simulink model "case8"  (R2024b)
settings: Solver=FixedStepAuto  StartTime=0  StopTime=1  FixedStep=1e-7  RelTol=1e-3
values from neighbouring files (symbols this model uses):
  SG_D_1_D = 0.01056    [IEEE9_case_parameters.m]    (also in case1_parameters.m; case2_parameters.m; case3_parameters.m; case4_parameters.m)
  SG_D_1_EnableSaturation = 0    [IEEE9_case_parameters.m]    (also in case1_parameters.m; case2_parameters.m; case3_parameters.m; case4_parameters.m)
  SG_D_1_f0 = 60    [IEEE9_case_parameters.m]    (also in case1_parameters.m; case2_parameters.m; case3_parameters.m; case4_parameters.m)
  SG_D_1_H = 7.5    [IEEE9_case_parameters.m]    (also in case1_parameters.m; case2_parameters.m; case3_parameters.m; case4_parameters.m)
  SG_D_1_K_A = 20    [IEEE9_case_parameters.m]    (also in case1_parameters.m; case2_parameters.m; case3_parameters.m; case4_parameters.m)
  SG_D_1_K_E = 1.000000e+1    (= 10)    [IEEE9_case_parameters.m]    (also in case1_parameters.m; case2_parameters.m; case3_parameters.m; case4_parameters.m)
  SG_D_1_K_F = 2.363    [IEEE9_case_parameters.m]    (also in case1_parameters.m; case2_parameters.m; case3_parameters.m; case4_parameters.m)
  SG_D_1_K_s = 0.5    [IEEE9_case_parameters.m]    (also in case1_parameters.m = 5; case2_parameters.m = 5; case3_parameters.m = 5; case4_parameters.m = 5)
  SG_D_1_R_a = 0.001088    [IEEE9_case_parameters.m]    (also in case1_parameters.m; case2_parameters.m; case3_parameters.m; case4_parameters.m)
  SG_D_1_S_A = 1    [IEEE9_case_parameters.m]    (also in case1_parameters.m; case2_parameters.m; case3_parameters.m; case4_parameters.m)
  SG_D_1_S_B = 0.103    [IEEE9_case_parameters.m]    (also in case1_parameters.m; case2_parameters.m; case3_parameters.m; case4_parameters.m)
  SG_D_1_S_N = 10.659857    [IEEE9_case_parameters.m]    (also in case1_parameters.m; case2_parameters.m; case3_parameters.m; case4_parameters.m)
  SG_D_1_SpeedPara = 200    [IEEE9_case_parameters.m]    (also in case1_parameters.m; case2_parameters.m; case3_parameters.m; case4_parameters.m)
  SG_D_1_T_0 = 0.720173    [IEEE9_case_parameters.m]    (also in case1_parameters.m = 0.755522; case2_parameters.m = 0.808931; case3_parameters.m = 0.869402; case4_parameters.m = 0.729316)
  SG_D_1_T_1 = 0.3    [IEEE9_case_parameters.m]    (also in case1_parameters.m; case2_parameters.m; case3_parameters.m; case4_parameters.m)
  SG_D_1_T_2 = 0.05    [IEEE9_case_parameters.m]    (also in case1_parameters.m; case2_parameters.m; case3_parameters.m; case4_parameters.m)
  SG_D_1_T_3 = 0.02    [IEEE9_case_parameters.m]    (also in case1_parameters.m; case2_parameters.m; case3_parameters.m; case4_parameters.m)
  SG_D_1_T_4 = 0.005    [IEEE9_case_parameters.m]    (also in case1_parameters.m; case2_parameters.m; case3_parameters.m; case4_parameters.m)
  SG_D_1_T_A = 0.02    [IEEE9_case_parameters.m]    (also in case1_parameters.m; case2_parameters.m; case3_parameters.m; case4_parameters.m)
  SG_D_1_T_dd = 8.000000e+0    (= 8)    [IEEE9_case_parameters.m]    (also in case1_parameters.m; case2_parameters.m; case3_parameters.m; case4_parameters.m)
  SG_D_1_T_ddd = 0.04    [IEEE9_case_parameters.m]    (also in case1_parameters.m; case2_parameters.m; case3_parameters.m; case4_parameters.m)
  SG_D_1_T_E = 0.314    [IEEE9_case_parameters.m]    (also in case1_parameters.m; case2_parameters.m; case3_parameters.m; case4_parameters.m)
  SG_D_1_T_F = 0.35    [IEEE9_case_parameters.m]    (also in case1_parameters.m; case2_parameters.m; case3_parameters.m; case4_parameters.m)
  SG_D_1_T_qd = 0.8    [IEEE9_case_parameters.m]    (also in case1_parameters.m; case2_parameters.m; case3_parameters.m; case4_parameters.m)
  SG_D_1_T_qdd = 0.02    [IEEE9_case_parameters.m]    (also in case1_parameters.m; case2_parameters.m; case3_parameters.m; case4_parameters.m)
  SG_D_1_T_speed = 0.1    [IEEE9_case_parameters.m]    (also in case1_parameters.m = 200; case2_parameters.m = 200; case3_parameters.m = 200; case4_parameters.m = 200)
  SG_D_1_T_w = 0.5    [IEEE9_case_parameters.m]    (also in case1_parameters.m; case2_parameters.m; case3_parameters.m; case4_parameters.m)
  SG_D_1_V_ref = 1.990276    [IEEE9_case_parameters.m]    (also in case1_parameters.m = 2.042296; case2_parameters.m = 2.051388; case3_parameters.m = 2.089584; case4_parameters.m = 2.01845)
  SG_D_1_w_ref = 376.991118    [IEEE9_case_parameters.m]    (also in case1_parameters.m; case2_parameters.m; case3_parameters.m; case4_parameters.m)
  SG_D_1_wb = 6.000000e+1    (= 60)    [IEEE9_case_parameters.m]    (also in case1_parameters.m; case2_parameters.m; case3_parameters.m; case4_parameters.m)
  SG_D_1_x_d = 1.9    [IEEE9_case_parameters.m]    (also in case1_parameters.m; case2_parameters.m; case3_parameters.m; case4_parameters.m)
  SG_D_1_x_dd = 0.302    [IEEE9_case_parameters.m]    (also in case1_parameters.m; case2_parameters.m; case3_parameters.m; case4_parameters.m)
  SG_D_1_x_ddd = 0.204    [IEEE9_case_parameters.m]    (also in case1_parameters.m; case2_parameters.m; case3_parameters.m; case4_parameters.m)
  SG_D_1_x_l = 0.05    [IEEE9_case_parameters.m]    (also in case1_parameters.m; case2_parameters.m; case3_parameters.m; case4_parameters.m)
  SG_D_1_x_q = 1.3    [IEEE9_case_parameters.m]    (also in case1_parameters.m; case2_parameters.m; case3_parameters.m; case4_parameters.m)
  SG_D_1_x_qd = 0.5    [IEEE9_case_parameters.m]    (also in case1_parameters.m; case2_parameters.m; case3_parameters.m; case4_parameters.m)
  SG_D_1_x_qdd = 0.3    [IEEE9_case_parameters.m]    (also in case1_parameters.m; case2_parameters.m; case3_parameters.m; case4_parameters.m)
  SG_D_2_D = 0.02    [IEEE9_case_parameters.m]    (also in case1_parameters.m; case2_parameters.m; case3_parameters.m; case4_parameters.m)
  SG_D_2_EnableSaturation = 0    [IEEE9_case_parameters.m]    (also in case1_parameters.m; case2_parameters.m; case3_parameters.m; case4_parameters.m)
  SG_D_2_f0 = 60    [IEEE9_case_parameters.m]    (also in case1_parameters.m; case2_parameters.m; case3_parameters.m; case4_parameters.m)
  SG_D_2_H = 8.000000e+0    (= 8)    [IEEE9_case_parameters.m]    (also in case1_parameters.m; case2_parameters.m; case3_parameters.m; case4_parameters.m)
  SG_D_2_K_A = 20    [IEEE9_case_parameters.m]    (also in case1_parameters.m; case2_parameters.m; case3_parameters.m; case4_parameters.m)
  SG_D_2_K_E = 1.000000e+1    (= 10)    [IEEE9_case_parameters.m]    (also in case1_parameters.m; case2_parameters.m; case3_parameters.m; case4_parameters.m)
  SG_D_2_K_F = 2.363    [IEEE9_case_parameters.m]    (also in case1_parameters.m; case2_parameters.m; case3_parameters.m; case4_parameters.m)
  SG_D_2_K_s = 0.5    [IEEE9_case_parameters.m]    (also in case1_parameters.m = 4; case2_parameters.m = 4; case3_parameters.m = 4; case4_parameters.m = 4)
  SG_D_2_R_a = 0.001088    [IEEE9_case_parameters.m]    (also in case1_parameters.m; case2_parameters.m; case3_parameters.m; case4_parameters.m)
  SG_D_2_S_A = 1    [IEEE9_case_parameters.m]    (also in case1_parameters.m; case2_parameters.m; case3_parameters.m; case4_parameters.m)
  SG_D_2_S_B = 0.103    [IEEE9_case_parameters.m]    (also in case1_parameters.m; case2_parameters.m; case3_parameters.m; case4_parameters.m)
  SG_D_2_S_N = 10.659857    [IEEE9_case_parameters.m]    (also in case1_parameters.m; case2_parameters.m; case3_parameters.m; case4_parameters.m)
  SG_D_2_SpeedPara = 200    [IEEE9_case_parameters.m]    (also in case1_parameters.m; case2_parameters.m; case3_parameters.m; case4_parameters.m)
  SG_D_2_T_0 = 1.632913    [IEEE9_case_parameters.m]    (also in case1_parameters.m = 1.632925; case2_parameters.m = 1.632915; case3_parameters.m = 1.632914; case4_parameters.m = 1.632927)
  SG_D_2_T_1 = 0.2    [IEEE9_case_parameters.m]    (also in case1_parameters.m; case2_parameters.m; case3_parameters.m; case4_parameters.m)
  SG_D_2_T_2 = 0.05    [IEEE9_case_parameters.m]    (also in case1_parameters.m; case2_parameters.m; case3_parameters.m; case4_parameters.m)
  SG_D_2_T_3 = 0.02    [IEEE9_case_parameters.m]    (also in case1_parameters.m; case2_parameters.m; case3_parameters.m; case4_parameters.m)
  SG_D_2_T_4 = 0.005    [IEEE9_case_parameters.m]    (also in case1_parameters.m; case2_parameters.m; case3_parameters.m; case4_parameters.m)
  SG_D_2_T_A = 0.02    [IEEE9_case_parameters.m]    (also in case1_parameters.m; case2_parameters.m; case3_parameters.m; case4_parameters.m)
  SG_D_2_T_dd = 7.9    [IEEE9_case_parameters.m]    (also in case1_parameters.m; case2_parameters.m; case3_parameters.m; case4_parameters.m)
  SG_D_2_T_ddd = 0.04    [IEEE9_case_parameters.m]    (also in case1_parameters.m; case2_parameters.m; case3_parameters.m; case4_parameters.m)
  SG_D_2_T_E = 0.314    [IEEE9_case_parameters.m]    (also in case1_parameters.m; case2_parameters.m; case3_parameters.m; case4_parameters.m)
  SG_D_2_T_F = 0.35    [IEEE9_case_parameters.m]    (also in case1_parameters.m; case2_parameters.m; case3_parameters.m; case4_parameters.m)
  SG_D_2_T_qd = 0.8    [IEEE9_case_parameters.m]    (also in case1_parameters.m; case2_parameters.m; case3_parameters.m; case4_parameters.m)
  SG_D_2_T_qdd = 0.015    [IEEE9_case_parameters.m]    (also in case1_parameters.m; case2_parameters.m; case3_parameters.m; case4_parameters.m)
  SG_D_2_T_speed = 0.1    [IEEE9_case_parameters.m]    (also in case1_parameters.m = 150; case2_parameters.m = 150; case3_parameters.m = 150; case4_parameters.m = 150)
  SG_D_2_T_w = 0.35    [IEEE9_case_parameters.m]    (also in case1_parameters.m; case2_parameters.m; case3_parameters.m; case4_parameters.m)
  SG_D_2_V_ref = 2.58547    [IEEE9_case_parameters.m]    (also in case1_parameters.m = 2.597896; case2_parameters.m = 2.587136; case3_parameters.m = 2.586042; case4_parameters.m = 2.599679)
  SG_D_2_w_ref = 376.991118    [IEEE9_case_parameters.m]    (also in case1_parameters.m; case2_parameters.m; case3_parameters.m; case4_parameters.m)
  SG_D_2_wb = 6.000000e+1    (= 60)    [IEEE9_case_parameters.m]    (also in case1_parameters.m; case2_parameters.m; case3_parameters.m; case4_parameters.m)
  SG_D_2_x_d = 1.8    [IEEE9_case_parameters.m]    (also in case1_parameters.m; case2_parameters.m; case3_parameters.m; case4_parameters.m)
  SG_D_2_x_dd = 0.302    [IEEE9_case_parameters.m]    (also in case1_parameters.m; case2_parameters.m; case3_parameters.m; case4_parameters.m)
  SG_D_2_x_ddd = 0.204    [IEEE9_case_parameters.m]    (also in case1_parameters.m; case2_parameters.m; case3_parameters.m; case4_parameters.m)
  SG_D_2_x_l = 0.05    [IEEE9_case_parameters.m]    (also in case1_parameters.m; case2_parameters.m; case3_parameters.m; case4_parameters.m)
  SG_D_2_x_q = 1.25    [IEEE9_case_parameters.m]    (also in case1_parameters.m; case2_parameters.m; case3_parameters.m; case4_parameters.m)
  SG_D_2_x_qd = 0.5    [IEEE9_case_parameters.m]    (also in case1_parameters.m; case2_parameters.m; case3_parameters.m; case4_parameters.m)
  SG_D_2_x_qdd = 0.3    [IEEE9_case_parameters.m]    (also in case1_parameters.m; case2_parameters.m; case3_parameters.m; case4_parameters.m)
  SG_D_3_D = 0.02    [IEEE9_case_parameters.m]    (also in case1_parameters.m; case2_parameters.m; case3_parameters.m; case4_parameters.m)
  SG_D_3_EnableSaturation = 0    [IEEE9_case_parameters.m]    (also in case1_parameters.m; case2_parameters.m; case3_parameters.m; case4_parameters.m)
  SG_D_3_f0 = 60    [IEEE9_case_parameters.m]    (also in case1_parameters.m; case2_parameters.m; case3_parameters.m; case4_parameters.m)
  SG_D_3_H = 7.7    [IEEE9_case_parameters.m]    (also in case1_parameters.m; case2_parameters.m; case3_parameters.m; case4_parameters.m)
  SG_D_3_K_A = 20    [IEEE9_case_parameters.m]    (also in case1_parameters.m; case2_parameters.m; case3_parameters.m; case4_parameters.m)
  SG_D_3_K_E = 1.000000e+1    (= 10)    [IEEE9_case_parameters.m]    (also in case1_parameters.m; case2_parameters.m; case3_parameters.m; case4_parameters.m)
  SG_D_3_K_F = 2.363    [IEEE9_case_parameters.m]    (also in case1_parameters.m; case2_parameters.m; case3_parameters.m; case4_parameters.m)
  SG_D_3_K_s = 0.2    [IEEE9_case_parameters.m]    (also in case1_parameters.m = 2; case2_parameters.m = 2; case3_parameters.m = 2; case4_parameters.m = 2)
  SG_D_3_R_a = 0.001088    [IEEE9_case_parameters.m]    (also in case1_parameters.m; case2_parameters.m; case3_parameters.m; case4_parameters.m)
  SG_D_3_S_A = 1    [IEEE9_case_parameters.m]    (also in case1_parameters.m; case2_parameters.m; case3_parameters.m; case4_parameters.m)
  SG_D_3_S_B = 0.103    [IEEE9_case_parameters.m]    (also in case1_parameters.m; case2_parameters.m; case3_parameters.m; case4_parameters.m)
  SG_D_3_S_N = 10.659857    [IEEE9_case_parameters.m]    (also in case1_parameters.m; case2_parameters.m; case3_parameters.m; case4_parameters.m)
  SG_D_3_SpeedPara = 200    [IEEE9_case_parameters.m]    (also in case1_parameters.m; case2_parameters.m; case3_parameters.m; case4_parameters.m)
  SG_D_3_T_0 = 0.850788    [IEEE9_case_parameters.m]    (also in case1_parameters.m = 0.850786; case2_parameters.m = 0.850787; case3_parameters.m; case4_parameters.m = 0.850786)
  SG_D_3_T_1 = 0.2    [IEEE9_case_parameters.m]    (also in case1_parameters.m; case2_parameters.m; case3_parameters.m; case4_parameters.m)
  SG_D_3_T_2 = 0.05    [IEEE9_case_parameters.m]    (also in case1_parameters.m; case2_parameters.m; case3_parameters.m; case4_parameters.m)
  SG_D_3_T_3 = 0.02    [IEEE9_case_parameters.m]    (also in case1_parameters.m; case2_parameters.m; case3_parameters.m; case4_parameters.m)
  SG_D_3_T_4 = 0.005    [IEEE9_case_parameters.m]    (also in case1_parameters.m; case2_parameters.m; case3_parameters.m; case4_parameters.m)
  SG_D_3_T_A = 0.02    [IEEE9_case_parameters.m]    (also in case1_parameters.m; case2_parameters.m; case3_parameters.m; case4_parameters.m)
  SG_D_3_T_dd = 8.1    [IEEE9_case_parameters.m]    (also in case1_parameters.m; case2_parameters.m; case3_parameters.m; case4_parameters.m)
  SG_D_3_T_ddd = 0.04    [IEEE9_case_parameters.m]    (also in case1_parameters.m; case2_parameters.m; case3_parameters.m; case4_parameters.m)
  SG_D_3_T_E = 0.314    [IEEE9_case_parameters.m]    (also in case1_parameters.m; case2_parameters.m; case3_parameters.m; case4_parameters.m)
  SG_D_3_T_F = 0.35    [IEEE9_case_parameters.m]    (also in case1_parameters.m; case2_parameters.m; case3_parameters.m; case4_parameters.m)
  SG_D_3_T_qd = 0.8    [IEEE9_case_parameters.m]    (also in case1_parameters.m; case2_parameters.m; case3_parameters.m; case4_parameters.m)
  SG_D_3_T_qdd = 0.015    [IEEE9_case_parameters.m]    (also in case1_parameters.m; case2_parameters.m; case3_parameters.m; case4_parameters.m)
  SG_D_3_T_speed = 0.1    [IEEE9_case_parameters.m]    (also in case1_parameters.m = 180; case2_parameters.m = 180; case3_parameters.m = 180; case4_parameters.m = 180)
  SG_D_3_T_w = 0.4    [IEEE9_case_parameters.m]    (also in case1_parameters.m; case2_parameters.m; case3_parameters.m; case4_parameters.m)
  SG_D_3_V_ref = 1.892727    [IEEE9_case_parameters.m]    (also in case1_parameters.m = 1.906439; case2_parameters.m = 1.895535; case3_parameters.m = 1.892105; case4_parameters.m = 1.906598)
  SG_D_3_w_ref = 376.991118    [IEEE9_case_parameters.m]    (also in case1_parameters.m; case2_parameters.m; case3_parameters.m; case4_parameters.m)
  SG_D_3_wb = 6.000000e+1    (= 60)    [IEEE9_case_parameters.m]    (also in case1_parameters.m; case2_parameters.m; case3_parameters.m; case4_parameters.m)
  SG_D_3_x_d = 1.85    [IEEE9_case_parameters.m]    (also in case1_parameters.m; case2_parameters.m; case3_parameters.m; case4_parameters.m)
  SG_D_3_x_dd = 0.302    [IEEE9_case_parameters.m]    (also in case1_parameters.m; case2_parameters.m; case3_parameters.m; case4_parameters.m)
  SG_D_3_x_ddd = 0.204    [IEEE9_case_parameters.m]    (also in case1_parameters.m; case2_parameters.m; case3_parameters.m; case4_parameters.m)
  SG_D_3_x_l = 0.05    [IEEE9_case_parameters.m]    (also in case1_parameters.m; case2_parameters.m; case3_parameters.m; case4_parameters.m)
  SG_D_3_x_q = 1.2    [IEEE9_case_parameters.m]    (also in case1_parameters.m; case2_parameters.m; case3_parameters.m; case4_parameters.m)
  SG_D_3_x_qd = 0.5    [IEEE9_case_parameters.m]    (also in case1_parameters.m; case2_parameters.m; case3_parameters.m; case4_parameters.m)
  SG_D_3_x_qdd = 0.3    [IEEE9_case_parameters.m]    (also in case1_parameters.m; case2_parameters.m; case3_parameters.m; case4_parameters.m)
(part 3 of 12)

== system case8/AC_1/d_id_load_7_block ==
  note: d_id_load_7 in case8
      | $376.991118430775\,\mathrm{iq}_{\mathrm{load},7}-1183.87051546095\,\mathrm{id}_{\mathrm{load},7}+1317.53755336093\,\mathrm{vd}_{\mathrm{bus},7}$
      | Automatically generated on 2025-10-31 19:30:30 .
  State_id_load_7_02c90 : Inport
  State_iq_load_7_8b7e4 : Inport  Port=2
  State_vd_bus_7_a966e : Inport  Port=3
  Add_4f71b : Sum
  Add_6d933 : Sum
  Constant_-1183.87051546095_9107f : Constant  Value=-1183.87051546095
  Constant_1317.53755336093_cc614 : Constant  Value=1317.53755336093
  Constant_376.991118430775_1b0b6 : Constant  Value=376.991118430775
  Product_0e383 : Product
  Product_2a875 : Product
  Product_da665 : Product
  Blockout_d_id_load_7_6563c : Outport
  wires:
  Constant_-1183.87051546095_9107f/1 -> Product_0e383/1
  Product_da665/1 -> Add_6d933/2
  State_id_load_7_02c90/1 -> Product_0e383/2
  Constant_376.991118430775_1b0b6/1 -> Product_da665/1
  Product_0e383/1 -> Add_6d933/1
  State_iq_load_7_8b7e4/1 -> Product_da665/2
  Constant_1317.53755336093_cc614/1 -> Product_2a875/1
  State_vd_bus_7_a966e/1 -> Product_2a875/2
  Add_6d933/1 -> Add_4f71b/1
  Product_2a875/1 -> Add_4f71b/2
  Add_4f71b/1 -> Blockout_d_id_load_7_6563c/1

== system case8/AC_1/d_id_load_9_block ==
  note: d_id_load_9 in case8
      | $376.991118430775\,\mathrm{iq}_{\mathrm{load},9}-1035.88670109407\,\mathrm{id}_{\mathrm{load},9}+1560.0268113928\,\mathrm{vd}_{\mathrm{bus},9}$
      | Automatically generated on 2025-10-31 19:30:31 .
  State_id_load_9_11d25 : Inport
  State_iq_load_9_fce7e : Inport  Port=2
  State_vd_bus_9_44d81 : Inport  Port=3
  Add_206f3 : Sum
  Add_ed7b0 : Sum
  Constant_-1035.88670109407_4e3e0 : Constant  Value=-1035.88670109407
  Constant_1560.0268113928_47ca8 : Constant  Value=1560.0268113928
  Constant_376.991118430775_fff66 : Constant  Value=376.991118430775
  Product_26dd0 : Product
  Product_89877 : Product
  Product_9ce91 : Product
  Blockout_d_id_load_9_27399 : Outport
  wires:
  Constant_-1035.88670109407_4e3e0/1 -> Product_26dd0/1
  Product_89877/1 -> Add_ed7b0/2
  State_id_load_9_11d25/1 -> Product_26dd0/2
  Constant_376.991118430775_fff66/1 -> Product_89877/1
  Product_26dd0/1 -> Add_ed7b0/1
  State_iq_load_9_fce7e/1 -> Product_89877/2
  Constant_1560.0268113928_47ca8/1 -> Product_9ce91/1
  State_vd_bus_9_44d81/1 -> Product_9ce91/2
  Add_ed7b0/1 -> Add_206f3/1
  Product_9ce91/1 -> Add_206f3/2
  Add_206f3/1 -> Blockout_d_id_load_9_27399/1

== system case8/AC_1/d_iq_line_1_4_block ==
  note: d_iq_line_1_4 in case8
      | $6464.71823947318\,\mathrm{vq}_{\mathrm{bus},1}-376.991118430775\,\mathrm{id}_{\mathrm{line},1,4}-6464.71823947318\,\mathrm{vq}_{\mathrm{bus},4}$
      | Automatically generated on 2025-10-31 19:30:32 .
  State_id_line_1_4_87a5d : Inport
  State_vq_bus_1_bc17e : Inport  Port=2
  State_vq_bus_4_19898 : Inport  Port=3
  Add_db077 : Sum
  Constant_-376.991118430775_442c6 : Constant  Value=-376.991118430775
  Constant_6464.71823947318_00242 : Constant  Value=6464.71823947318
  Constant_6464.71823947318_50f7c : Constant  Value=6464.71823947318
  Product_53a87 : Product
  Product_6dd1f : Product
  Product_bbc40 : Product
  Subtract_23de6 : Sum  Inputs=+-
  Blockout_d_iq_line_1_4_90247 : Outport
  wires:
  Constant_-376.991118430775_442c6/1 -> Product_53a87/1
  Product_bbc40/1 -> Add_db077/2
  State_id_line_1_4_87a5d/1 -> Product_53a87/2
  Constant_6464.71823947318_00242/1 -> Product_bbc40/1
  Product_53a87/1 -> Add_db077/1
  Subtract_23de6/1 -> Blockout_d_iq_line_1_4_90247/1
  State_vq_bus_1_bc17e/1 -> Product_bbc40/2
  Constant_6464.71823947318_50f7c/1 -> Product_6dd1f/1
  State_vq_bus_4_19898/1 -> Product_6dd1f/2
  Add_db077/1 -> Subtract_23de6/1
  Product_6dd1f/1 -> Subtract_23de6/2

== system case8/AC_1/d_iq_line_3_6_block ==
  note: d_iq_line_3_6 in case8
      | $6354.39881559139\,\mathrm{vq}_{\mathrm{bus},3}-376.991118430775\,\mathrm{id}_{\mathrm{line},3,6}-6354.39881559139\,\mathrm{vq}_{\mathrm{bus},6}$
      | Automatically generated on 2025-10-31 19:30:34 .
  State_id_line_3_6_2080e : Inport
  State_vq_bus_3_4f015 : Inport  Port=2
  State_vq_bus_6_02815 : Inport  Port=3
  Add_778b1 : Sum
  Constant_-376.991118430775_aab41 : Constant  Value=-376.991118430775
  Constant_6354.39881559139_a9d77 : Constant  Value=6354.39881559139
  Constant_6354.39881559139_c319a : Constant  Value=6354.39881559139
  Product_e1a54 : Product
  Product_e93f9 : Product
  Product_f50dd : Product
  Subtract_8e4b8 : Sum  Inputs=+-
  Blockout_d_iq_line_3_6_dcf40 : Outport
  wires:
  Constant_-376.991118430775_aab41/1 -> Product_e1a54/1
  Product_e93f9/1 -> Add_778b1/2
  State_id_line_3_6_2080e/1 -> Product_e1a54/2
  Constant_6354.39881559139_c319a/1 -> Product_e93f9/1
  Product_e1a54/1 -> Add_778b1/1
  State_vq_bus_3_4f015/1 -> Product_e93f9/2
  Constant_6354.39881559139_a9d77/1 -> Product_f50dd/1
  State_vq_bus_6_02815/1 -> Product_f50dd/2
  Add_778b1/1 -> Subtract_8e4b8/1
  Product_f50dd/1 -> Subtract_8e4b8/2
  Subtract_8e4b8/1 -> Blockout_d_iq_line_3_6_dcf40/1

== system case8/AC_1/d_iq_line_4_5_block ==
  note: d_iq_line_4_5 in case8
      | $4047.47576732234\,\mathrm{vq}_{\mathrm{bus},4}-64.2696492842669\,\mathrm{iq}_{\mathrm{line},4,5}-376.991118430775\,\mathrm{id}_{\mathrm{line},4,5}-4047.47576732234\,\mathrm{vq}_{\mathrm{bus},5}$
      | Automatically generated on 2025-10-31 19:30:33 .
  State_id_line_4_5_e9364 : Inport
  State_iq_line_4_5_eb553 : Inport  Port=2
  State_vq_bus_4_c7938 : Inport  Port=3
  State_vq_bus_5_05939 : Inport  Port=4
  Add_c346b : Sum
  Constant_-376.991118430775_d5068 : Constant  Value=-376.991118430775
  Constant_4047.47576732234_74ae1 : Constant  Value=4047.47576732234
  Constant_4047.47576732234_942cd : Constant  Value=4047.47576732234
  Constant_64.2696492842669_2e641 : Constant  Value=64.2696492842669
  Product_4e02b : Product
  Product_70603 : Product
  Product_c244d : Product
  Product_d87fe : Product
  Subtract_71308 : Sum  Inputs=+-
  Subtract_83d8f : Sum  Inputs=+-
  Blockout_d_iq_line_4_5_40906 : Outport
  wires:
  Constant_-376.991118430775_d5068/1 -> Product_4e02b/1
  Constant_64.2696492842669_2e641/1 -> Product_c244d/1
  State_id_line_4_5_e9364/1 -> Product_4e02b/2
  State_iq_line_4_5_eb553/1 -> Product_c244d/2
  Product_4e02b/1 -> Subtract_71308/1
  Constant_4047.47576732234_942cd/1 -> Product_70603/1
  Product_c244d/1 -> Subtract_71308/2
  State_vq_bus_4_c7938/1 -> Product_70603/2
  Subtract_71308/1 -> Add_c346b/1
  Product_70603/1 -> Add_c346b/2
  Constant_4047.47576732234_74ae1/1 -> Product_d87fe/1
  State_vq_bus_5_05939/1 -> Product_d87fe/2
  Add_c346b/1 -> Subtract_83d8f/1
  Product_d87fe/1 -> Subtract_83d8f/2
  Subtract_83d8f/1 -> Blockout_d_iq_line_4_5_40906/1

== system case8/AC_1/d_iq_line_5_6_block ==
  note: d_iq_line_5_6 in case8
      | $2190.39865055091\,\mathrm{vq}_{\mathrm{bus},5}-79.7922150975604\,\mathrm{iq}_{\mathrm{line},5,6}-376.991118430775\,\mathrm{id}_{\mathrm{line},5,6}-2190.39865055091\,\mathrm{vq}_{\mathrm{bus},6}$
      | Automatically generated on 2025-10-31 19:30:34 .
  State_id_line_5_6_be082 : Inport
  State_iq_line_5_6_a09e9 : Inport  Port=2
  State_vq_bus_5_af966 : Inport  Port=3
  State_vq_bus_6_d8e58 : Inport  Port=4
  Add_b20bd : Sum
  Constant_-376.991118430775_2cd5f : Constant  Value=-376.991118430775
  Constant_2190.39865055091_98720 : Constant  Value=2190.39865055091
  Constant_2190.39865055091_cee28 : Constant  Value=2190.39865055091
  Constant_79.7922150975604_67a7c : Constant  Value=79.7922150975604
  Product_21308 : Product
  Product_25905 : Product
  Product_4c5a0 : Product
  Product_8b4be : Product
  Subtract_12dc3 : Sum  Inputs=+-
  Subtract_5257b : Sum  Inputs=+-
  Blockout_d_iq_line_5_6_2f920 : Outport
  wires:
  Constant_-376.991118430775_2cd5f/1 -> Product_21308/1
  Constant_79.7922150975604_67a7c/1 -> Product_4c5a0/1
  Subtract_12dc3/1 -> Blockout_d_iq_line_5_6_2f920/1
  State_id_line_5_6_be082/1 -> Product_21308/2
  State_iq_line_5_6_a09e9/1 -> Product_4c5a0/2
  Product_21308/1 -> Subtract_5257b/1
  Constant_2190.39865055091_cee28/1 -> Product_8b4be/1
  Product_4c5a0/1 -> Subtract_5257b/2
  Product_25905/1 -> Subtract_12dc3/2
  State_vq_bus_5_af966/1 -> Product_8b4be/2
  Subtract_5257b/1 -> Add_b20bd/1
  Product_8b4be/1 -> Add_b20bd/2
  Constant_2190.39865055091_98720/1 -> Product_25905/1
  State_vq_bus_6_d8e58/1 -> Product_25905/2
  Add_b20bd/1 -> Subtract_12dc3/1

== system case8/AC_1/d_iq_line_6_7_block ==
  note: d_iq_line_6_7 in case8
      | $3694.12470827039\,\mathrm{vq}_{\mathrm{bus},6}-41.0611648205039\,\mathrm{iq}_{\mathrm{line},6,7}-376.991118430775\,\mathrm{id}_{\mathrm{line},6,7}-3694.12470827039\,\mathrm{vq}_{\mathrm{bus},7}$
      | Automatically generated on 2025-10-31 19:30:35 .
  State_id_line_6_7_9c15a : Inport
  State_iq_line_6_7_14306 : Inport  Port=2
  State_vq_bus_6_bc18e : Inport  Port=3
  State_vq_bus_7_61479 : Inport  Port=4
  Add_9131e : Sum
  Constant_-376.991118430775_1a441 : Constant  Value=-376.991118430775
  Constant_3694.12470827039_28c0b : Constant  Value=3694.12470827039
  Constant_3694.12470827039_ad879 : Constant  Value=3694.12470827039
  Constant_41.0611648205039_0ab7d : Constant  Value=41.0611648205039
  Product_00459 : Product
  Product_1ddd6 : Product
  Product_1dfdc : Product
  Product_dca75 : Product
  Subtract_45c2b : Sum  Inputs=+-
  Subtract_615ba : Sum  Inputs=+-
  Blockout_d_iq_line_6_7_91852 : Outport
  wires:
  Constant_-376.991118430775_1a441/1 -> Product_00459/1
  Constant_41.0611648205039_0ab7d/1 -> Product_dca75/1
  State_id_line_6_7_9c15a/1 -> Product_00459/2
  State_iq_line_6_7_14306/1 -> Product_dca75/2
  Product_00459/1 -> Subtract_45c2b/1
  Constant_3694.12470827039_ad879/1 -> Product_1ddd6/1
  Product_dca75/1 -> Subtract_45c2b/2
  State_vq_bus_6_bc18e/1 -> Product_1ddd6/2
  Subtract_45c2b/1 -> Add_9131e/1
  Product_1ddd6/1 -> Add_9131e/2
  Constant_3694.12470827039_28c0b/1 -> Product_1dfdc/1
  State_vq_bus_7_61479/1 -> Product_1dfdc/2
  Add_9131e/1 -> Subtract_615ba/1
  Product_1dfdc/1 -> Subtract_615ba/2
  Subtract_615ba/1 -> Blockout_d_iq_line_6_7_91852/1

== system case8/AC_1/d_iq_line_7_8_block ==
  note: d_iq_line_7_8 in case8
      | $5171.77459157855\,\mathrm{vq}_{\mathrm{bus},7}-41.0611648205039\,\mathrm{iq}_{\mathrm{line},7,8}-376.991118430775\,\mathrm{id}_{\mathrm{line},7,8}-5171.77459157855\,\mathrm{vq}_{\mathrm{bus},8}$
      | Automatically generated on 2025-10-31 19:30:36 .
  State_id_line_7_8_e4da3 : Inport
  State_iq_line_7_8_8ce3b : Inport  Port=2
  State_vq_bus_7_e4b2c : Inport  Port=3
  State_vq_bus_8_f3b64 : Inport  Port=4
  Add_a5f94 : Sum
  Constant_-376.991118430775_b9f31 : Constant  Value=-376.991118430775
  Constant_41.0611648205039_094c3 : Constant  Value=41.0611648205039
  Constant_5171.77459157855_4f937 : Constant  Value=5171.77459157855
  Constant_5171.77459157855_f8443 : Constant  Value=5171.77459157855
  Product_091ec : Product
  Product_8188b : Product
  Product_9f885 : Product
  Product_e30da : Product
  Subtract_21a37 : Sum  Inputs=+-
  Subtract_723c1 : Sum  Inputs=+-
  Blockout_d_iq_line_7_8_2e847 : Outport
  wires:
  Constant_-376.991118430775_b9f31/1 -> Product_091ec/1
  Constant_41.0611648205039_094c3/1 -> Product_8188b/1
  State_id_line_7_8_e4da3/1 -> Product_091ec/2
  State_iq_line_7_8_8ce3b/1 -> Product_8188b/2
  Product_091ec/1 -> Subtract_21a37/1
  Constant_5171.77459157855_f8443/1 -> Product_e30da/1
  Product_8188b/1 -> Subtract_21a37/2
  State_vq_bus_7_e4b2c/1 -> Product_e30da/2
  Subtract_21a37/1 -> Add_a5f94/1
  Product_e30da/1 -> Add_a5f94/2
  Constant_5171.77459157855_4f937/1 -> Product_9f885/1
  State_vq_bus_8_f3b64/1 -> Product_9f885/2
  Add_a5f94/1 -> Subtract_723c1/1
  Product_9f885/1 -> Subtract_723c1/2
  Subtract_723c1/1 -> Blockout_d_iq_line_7_8_2e847/1

== system case8/AC_1/d_iq_line_8_2_block ==
  note: d_iq_line_8_2 in case8
      | $5957.88432949849\,\mathrm{vq}_{\mathrm{bus},8}-5957.88432949849\,\mathrm{vq}_{\mathrm{bus},2}-376.991118430775\,\mathrm{id}_{\mathrm{line},8,2}$
      | Automatically generated on 2025-10-31 19:30:37 .
  State_id_line_8_2_40f60 : Inport
  State_vq_bus_2_064cf : Inport  Port=2
  State_vq_bus_8_f7efd : Inport  Port=3
  Add_4063f : Sum
  Constant_-376.991118430775_1a7d4 : Constant  Value=-376.991118430775
  Constant_5957.88432949849_649d9 : Constant  Value=5957.88432949849
  Constant_5957.88432949849_cf729 : Constant  Value=5957.88432949849
  Product_09a3a : Product
  Product_ca0c4 : Product
  Product_f6dd3 : Product
  Subtract_b9b6e : Sum  Inputs=+-
  Blockout_d_iq_line_8_2_f14cf : Outport
  wires:
  Constant_-376.991118430775_1a7d4/1 -> Product_ca0c4/1
  Product_09a3a/1 -> Subtract_b9b6e/2
  State_id_line_8_2_40f60/1 -> Product_ca0c4/2
  Constant_5957.88432949849_649d9/1 -> Product_09a3a/1
  Product_ca0c4/1 -> Subtract_b9b6e/1
  State_vq_bus_2_064cf/1 -> Product_09a3a/2
  Constant_5957.88432949849_cf729/1 -> Product_f6dd3/1
  State_vq_bus_8_f7efd/1 -> Product_f6dd3/2
  Subtract_b9b6e/1 -> Add_4063f/1
  Product_f6dd3/1 -> Add_4063f/2
  Add_4063f/1 -> Blockout_d_iq_line_8_2_f14cf/1

== system case8/AC_1/d_iq_line_8_9_block ==
  note: d_iq_line_8_9 in case8
      | $2312.84329561277\,\mathrm{vq}_{\mathrm{bus},8}-69.1303790620686\,\mathrm{iq}_{\mathrm{line},8,9}-376.991118430775\,\mathrm{id}_{\mathrm{line},8,9}-2312.84329561277\,\mathrm{vq}_{\mathrm{bus},9}$
      | Automatically generated on 2025-10-31 19:30:38 .
  State_id_line_8_9_e905c : Inport
  State_iq_line_8_9_3bed7 : Inport  Port=2
  State_vq_bus_8_e6dc9 : Inport  Port=3
  State_vq_bus_9_10dc5 : Inport  Port=4
  Add_a305c : Sum
  Constant_-376.991118430775_3d292 : Constant  Value=-376.991118430775
  Constant_2312.84329561277_b2070 : Constant  Value=2312.84329561277
  Constant_2312.84329561277_e4d87 : Constant  Value=2312.84329561277
  Constant_69.1303790620686_84fc2 : Constant  Value=69.1303790620686
  Product_39918 : Product
  Product_706d2 : Product
  Product_96cf0 : Product
  Product_d7411 : Product
  Subtract_3fa01 : Sum  Inputs=+-
  Subtract_d9459 : Sum  Inputs=+-
  Blockout_d_iq_line_8_9_9da92 : Outport
  wires:
  Constant_-376.991118430775_3d292/1 -> Product_d7411/1
  Constant_69.1303790620686_84fc2/1 -> Product_706d2/1
  State_id_line_8_9_e905c/1 -> Product_d7411/2
  State_iq_line_8_9_3bed7/1 -> Product_706d2/2
  Product_d7411/1 -> Subtract_d9459/1
  Constant_2312.84329561277_b2070/1 -> Product_39918/1
  Product_706d2/1 -> Subtract_d9459/2
  State_vq_bus_8_e6dc9/1 -> Product_39918/2
  Subtract_d9459/1 -> Add_a305c/1
  Product_39918/1 -> Add_a305c/2
  Constant_2312.84329561277_e4d87/1 -> Product_96cf0/1
  Add_a305c/1 -> Subtract_3fa01/1
  State_vq_bus_9_10dc5/1 -> Product_96cf0/2
  Product_96cf0/1 -> Subtract_3fa01/2
  Subtract_3fa01/1 -> Blockout_d_iq_line_8_9_9da92/1

== system case8/AC_1/d_iq_line_9_4_block ==
  note: d_iq_line_9_4 in case8
      | $4380.79730110183\,\mathrm{vq}_{\mathrm{bus},9}-40.9190846654156\,\mathrm{iq}_{\mathrm{line},9,4}-4380.79730110183\,\mathrm{vq}_{\mathrm{bus},4}-376.991118430775\,\mathrm{id}_{\mathrm{line},9,4}$
      | Automatically generated on 2025-10-31 19:30:39 .
  State_id_line_9_4_0b3a3 : Inport
  State_iq_line_9_4_e794a : Inport  Port=2
  State_vq_bus_4_b5a4c : Inport  Port=3
  State_vq_bus_9_b8c36 : Inport  Port=4
  Add_dd79f : Sum
  Constant_-376.991118430775_ef531 : Constant  Value=-376.991118430775
  Constant_40.9190846654156_15435 : Constant  Value=40.9190846654156
  Constant_4380.79730110183_865ff : Constant  Value=4380.79730110183
  Constant_4380.79730110183_a4a98 : Constant  Value=4380.79730110183
  Product_004cb : Product
  Product_1ebe1 : Product
  Product_909ca : Product
  Product_e1a86 : Product
  Subtract_0b837 : Sum  Inputs=+-
  Subtract_7e3de : Sum  Inputs=+-
  Blockout_d_iq_line_9_4_17728 : Outport
  wires:
  Constant_-376.991118430775_ef531/1 -> Product_909ca/1
  Constant_40.9190846654156_15435/1 -> Product_1ebe1/1
  State_id_line_9_4_0b3a3/1 -> Product_909ca/2
  State_iq_line_9_4_e794a/1 -> Product_1ebe1/2
  Product_909ca/1 -> Subtract_7e3de/1
  Constant_4380.79730110183_a4a98/1 -> Product_e1a86/1
  Product_1ebe1/1 -> Subtract_7e3de/2
  State_vq_bus_4_b5a4c/1 -> Product_e1a86/2
  Subtract_7e3de/1 -> Subtract_0b837/1
  Product_e1a86/1 -> Subtract_0b837/2
  Constant_4380.79730110183_865ff/1 -> Product_004cb/1
  Add_dd79f/1 -> Blockout_d_iq_line_9_4_17728/1
  State_vq_bus_9_b8c36/1 -> Product_004cb/2
  Subtract_0b837/1 -> Add_dd79f/1
  Product_004cb/1 -> Add_dd79f/2

== system case8/AC_1/d_iq_load_5_block ==
  note: d_iq_load_5 in case8
      | $1255.7149080224\,\mathrm{vq}_{\mathrm{bus},5}-1243.06404152488\,\mathrm{iq}_{\mathrm{load},5}-376.991118430775\,\mathrm{id}_{\mathrm{load},5}$
      | Automatically generated on 2025-10-31 19:30:29 .
  State_id_load_5_6ba41 : Inport
  State_iq_load_5_f938b : Inport  Port=2
  State_vq_bus_5_44727 : Inport  Port=3
  Add_81567 : Sum
  Constant_-376.991118430775_6218a : Constant  Value=-376.991118430775
  Constant_1243.06404152488_c11a3 : Constant  Value=1243.06404152488
  Constant_1255.7149080224_8070c : Constant  Value=1255.7149080224
  Product_3828c : Product
  Product_38469 : Product
  Product_8c4e0 : Product
  Subtract_501d6 : Sum  Inputs=+-
  Blockout_d_iq_load_5_439b9 : Outport
  wires:
  Constant_-376.991118430775_6218a/1 -> Product_3828c/1
  Product_8c4e0/1 -> Subtract_501d6/2
  State_id_load_5_6ba41/1 -> Product_3828c/2
  Constant_1243.06404152488_c11a3/1 -> Product_8c4e0/1
  Product_3828c/1 -> Subtract_501d6/1
  State_iq_load_5_f938b/1 -> Product_8c4e0/2
  Constant_1255.7149080224_8070c/1 -> Product_38469/1
  State_vq_bus_5_44727/1 -> Product_38469/2
  Subtract_501d6/1 -> Add_81567/1
  Product_38469/1 -> Add_81567/2
  Add_81567/1 -> Blockout_d_iq_load_5_439b9/1

== system case8/AC_1/d_iq_load_7_block ==
  note: d_iq_load_7 in case8
      | $1317.53755336093\,\mathrm{vq}_{\mathrm{bus},7}-1183.87051546095\,\mathrm{iq}_{\mathrm{load},7}-376.991118430775\,\mathrm{id}_{\mathrm{load},7}$
      | Automatically generated on 2025-10-31 19:30:30 .
  State_id_load_7_0f4df : Inport
  State_iq_load_7_d963a : Inport  Port=2
  State_vq_bus_7_cd2e6 : Inport  Port=3
  Add_e526c : Sum
  Constant_-376.991118430775_0eb74 : Constant  Value=-376.991118430775
  Constant_1183.87051546095_5bd87 : Constant  Value=1183.87051546095
  Constant_1317.53755336093_5e011 : Constant  Value=1317.53755336093
  Product_0ead2 : Product
  Product_a75ff : Product
  Product_bbb39 : Product
  Subtract_ba69a : Sum  Inputs=+-
  Blockout_d_iq_load_7_3ba97 : Outport
  wires:
  Constant_-376.991118430775_0eb74/1 -> Product_0ead2/1
  Product_bbb39/1 -> Subtract_ba69a/2
  State_id_load_7_0f4df/1 -> Product_0ead2/2
  Constant_1183.87051546095_5bd87/1 -> Product_bbb39/1
  Product_0ead2/1 -> Subtract_ba69a/1
  State_iq_load_7_d963a/1 -> Product_bbb39/2
  Constant_1317.53755336093_5e011/1 -> Product_a75ff/1
  State_vq_bus_7_cd2e6/1 -> Product_a75ff/2
  Subtract_ba69a/1 -> Add_e526c/1
  Product_a75ff/1 -> Add_e526c/2
  Add_e526c/1 -> Blockout_d_iq_load_7_3ba97/1

== system case8/AC_1/d_iq_load_9_block ==
  note: d_iq_load_9 in case8
      | $1560.0268113928\,\mathrm{vq}_{\mathrm{bus},9}-1035.88670109407\,\mathrm{iq}_{\mathrm{load},9}-376.991118430775\,\mathrm{id}_{\mathrm{load},9}$
      | Automatically generated on 2025-10-31 19:30:31 .
  State_id_load_9_21d1c : Inport
  State_iq_load_9_9492a : Inport  Port=2
  State_vq_bus_9_325e9 : Inport  Port=3
  Add_7d0d5 : Sum
  Constant_-376.991118430775_b5781 : Constant  Value=-376.991118430775
  Constant_1035.88670109407_adb08 : Constant  Value=1035.88670109407
  Constant_1560.0268113928_e99c5 : Constant  Value=1560.0268113928
  Product_0e898 : Product
  Product_752c8 : Product
  Product_a0f2f : Product
  Subtract_df731 : Sum  Inputs=+-
  Blockout_d_iq_load_9_3eba4 : Outport
  wires:
  Constant_-376.991118430775_b5781/1 -> Product_0e898/1
  Product_752c8/1 -> Subtract_df731/2
  State_id_load_9_21d1c/1 -> Product_0e898/2
  Add_7d0d5/1 -> Blockout_d_iq_load_9_3eba4/1
  Constant_1035.88670109407_adb08/1 -> Product_752c8/1
  Product_a0f2f/1 -> Add_7d0d5/2
  Product_0e898/1 -> Subtract_df731/1
  State_iq_load_9_9492a/1 -> Product_752c8/2
  Constant_1560.0268113928_e99c5/1 -> Product_a0f2f/1
  State_vq_bus_9_325e9/1 -> Product_a0f2f/2
  Subtract_df731/1 -> Add_7d0d5/1

== system case8/AC_1/d_vd_bus_1_block ==
  note: d_vd_bus_1 in case8
      | $37699111.8430775\,\mathrm{id}_{\mathrm{bus},1}+376.991118430775\,\mathrm{vq}_{\mathrm{bus},1}$
      | Automatically generated on 2025-10-31 19:30:25 .
  Alge_id_bus_1_2d668 : Inport
  State_vq_bus_1_4702e : Inport  Port=2
  Add_27c1b : Sum
  Constant_376.991118430775_16303 : Constant  Value=376.991118430775
  Constant_37699111.8430775_9dade : Constant  Value=37699111.8430775
  Product_7ead7 : Product
  Product_fb150 : Product
  Blockout_d_vd_bus_1_b1cc3 : Outport
  wires:
  Constant_37699111.8430775_9dade/1 -> Product_fb150/1
  Product_7ead7/1 -> Add_27c1b/2
  Alge_id_bus_1_2d668/1 -> Product_fb150/2
  Constant_376.991118430775_16303/1 -> Product_7ead7/1
  State_vq_bus_1_4702e/1 -> Product_7ead7/2
  Add_27c1b/1 -> Blockout_d_vd_bus_1_b1cc3/1
  Product_fb150/1 -> Add_27c1b/1

== system case8/AC_1/d_vd_bus_2_block ==
  note: d_vd_bus_2 in case8
      | $37699111.8430775\,\mathrm{id}_{\mathrm{bus},2}+376.991118430775\,\mathrm{vq}_{\mathrm{bus},2}$
      | Automatically generated on 2025-10-31 19:30:25 .
  Alge_id_bus_2_5a7f8 : Inport
  State_vq_bus_2_9c28c : Inport  Port=2
  Add_67458 : Sum
  Constant_376.991118430775_dacd7 : Constant  Value=376.991118430775
  Constant_37699111.8430775_48296 : Constant  Value=37699111.8430775
  Product_cad1b : Product
  Product_d6b91 : Product
  Blockout_d_vd_bus_2_136aa : Outport
  wires:
  Constant_37699111.8430775_48296/1 -> Product_cad1b/1
  Product_d6b91/1 -> Add_67458/2
  Alge_id_bus_2_5a7f8/1 -> Product_cad1b/2
  Constant_376.991118430775_dacd7/1 -> Product_d6b91/1
  Product_cad1b/1 -> Add_67458/1
  State_vq_bus_2_9c28c/1 -> Product_d6b91/2
  Add_67458/1 -> Blockout_d_vd_bus_2_136aa/1

== system case8/AC_1/d_vd_bus_3_block ==
  note: d_vd_bus_3 in case8
      | $37699111.8430775\,\mathrm{id}_{\mathrm{bus},3}+376.991118430775\,\mathrm{vq}_{\mathrm{bus},3}$
      | Automatically generated on 2025-10-31 19:30:26 .
  Alge_id_bus_3_24e35 : Inport
  State_vq_bus_3_73cd2 : Inport  Port=2
  Add_687c4 : Sum
  Constant_376.991118430775_06d9e : Constant  Value=376.991118430775
  Constant_37699111.8430775_24c42 : Constant  Value=37699111.8430775
  Product_146a7 : Product
  Product_a9927 : Product
  Blockout_d_vd_bus_3_5ac98 : Outport
  wires:
  Constant_37699111.8430775_24c42/1 -> Product_146a7/1
  Product_a9927/1 -> Add_687c4/2
  Alge_id_bus_3_24e35/1 -> Product_146a7/2
  Constant_376.991118430775_06d9e/1 -> Product_a9927/1
  Product_146a7/1 -> Add_687c4/1
  State_vq_bus_3_73cd2/1 -> Product_a9927/2
  Add_687c4/1 -> Blockout_d_vd_bus_3_5ac98/1

== system case8/AC_1/d_vd_bus_4_block ==
  note: d_vd_bus_4 in case8
      | $2257.43184689087\,\mathrm{id}_{\mathrm{bus},4}+376.991118430775\,\mathrm{vq}_{\mathrm{bus},4}$
      | Automatically generated on 2025-10-31 19:30:26 .
  Alge_id_bus_4_17e21 : Inport
  State_vq_bus_4_796f6 : Inport  Port=2
  Add_3847a : Sum
  Constant_2257.43184689087_f1eca : Constant  Value=2257.43184689087
  Constant_376.991118430775_94836 : Constant  Value=376.991118430775
  Product_744e0 : Product
  Product_d80c4 : Product
  Blockout_d_vd_bus_4_449c0 : Outport
  wires:
  Constant_2257.43184689087_f1eca/1 -> Product_d80c4/1
  Product_744e0/1 -> Add_3847a/2
  Alge_id_bus_4_17e21/1 -> Product_d80c4/2
  Constant_376.991118430775_94836/1 -> Product_744e0/1
  Product_d80c4/1 -> Add_3847a/1
  State_vq_bus_4_796f6/1 -> Product_744e0/2
  Add_3847a/1 -> Blockout_d_vd_bus_4_449c0/1

== system case8/AC_1/d_vd_bus_5_block ==
  note: d_vd_bus_5 in case8
      | $1461.2058853906\,\mathrm{id}_{\mathrm{bus},5}+376.991118430775\,\mathrm{vq}_{\mathrm{bus},5}$
      | Automatically generated on 2025-10-31 19:30:27 .
  Alge_id_bus_5_9ae33 : Inport
  State_vq_bus_5_87df7 : Inport  Port=2
  Add_56656 : Sum
  Constant_1461.2058853906_c6dd8 : Constant  Value=1461.2058853906
  Constant_376.991118430775_070e5 : Constant  Value=376.991118430775
  Product_1cb87 : Product
  Product_2475c : Product
  Blockout_d_vd_bus_5_3f620 : Outport
  wires:
  Constant_1461.2058853906_c6dd8/1 -> Product_1cb87/1
  Product_2475c/1 -> Add_56656/2
  Alge_id_bus_5_9ae33/1 -> Product_1cb87/2
  Constant_376.991118430775_070e5/1 -> Product_2475c/1
  Product_1cb87/1 -> Add_56656/1
  State_vq_bus_5_87df7/1 -> Product_2475c/2
  Add_56656/1 -> Blockout_d_vd_bus_5_3f620/1

== system case8/AC_1/d_vd_bus_6_block ==
  note: d_vd_bus_6 in case8
      | $1329.77466818616\,\mathrm{id}_{\mathrm{bus},6}+376.991118430775\,\mathrm{vq}_{\mathrm{bus},6}$
      | Automatically generated on 2025-10-31 19:30:27 .
  Alge_id_bus_6_c988e : Inport
  State_vq_bus_6_96ef6 : Inport  Port=2
  Add_2b2df : Sum
  Constant_1329.77466818616_db93a : Constant  Value=1329.77466818616
  Constant_376.991118430775_a189c : Constant  Value=376.991118430775
  Product_6f5a4 : Product
  Product_7baa2 : Product
  Blockout_d_vd_bus_6_cfd11 : Outport
  wires:
  Constant_1329.77466818616_db93a/1 -> Product_6f5a4/1
  Product_7baa2/1 -> Add_2b2df/2
  Alge_id_bus_6_c988e/1 -> Product_6f5a4/2
  Constant_376.991118430775_a189c/1 -> Product_7baa2/1
  Product_6f5a4/1 -> Add_2b2df/1
  State_vq_bus_6_96ef6/1 -> Product_7baa2/2
  Add_2b2df/1 -> Blockout_d_vd_bus_6_cfd11/1

== system case8/AC_1/d_vd_bus_7_block ==
  note: d_vd_bus_7 in case8
      | $2106.09563369148\,\mathrm{id}_{\mathrm{bus},7}+376.991118430775\,\mathrm{vq}_{\mathrm{bus},7}$
      | Automatically generated on 2025-10-31 19:30:28 .
  Alge_id_bus_7_9e4a6 : Inport
  State_vq_bus_7_fd391 : Inport  Port=2
  Add_e127f : Sum
  Constant_2106.09563369148_e2a0b : Constant  Value=2106.09563369148
  Constant_376.991118430775_17e76 : Constant  Value=376.991118430775
  Product_3a5bd : Product
  Product_c7cc5 : Product
  Blockout_d_vd_bus_7_43381 : Outport
  wires:
  Constant_2106.09563369148_e2a0b/1 -> Product_3a5bd/1
  Product_c7cc5/1 -> Add_e127f/2
  Alge_id_bus_7_9e4a6/1 -> Product_3a5bd/2
  Constant_376.991118430775_17e76/1 -> Product_c7cc5/1
  Product_3a5bd/1 -> Add_e127f/1
  State_vq_bus_7_fd391/1 -> Product_c7cc5/2
  Add_e127f/1 -> Blockout_d_vd_bus_7_43381/1

== system case8/AC_1/d_vd_bus_8_block ==
  note: d_vd_bus_8 in case8
      | $1657.10381727813\,\mathrm{id}_{\mathrm{bus},8}+376.991118430775\,\mathrm{vq}_{\mathrm{bus},8}$
      | Automatically generated on 2025-10-31 19:30:28 .
  Alge_id_bus_8_8b650 : Inport
  State_vq_bus_8_643ce : Inport  Port=2
  Add_698bd : Sum
  Constant_1657.10381727813_58e15 : Constant  Value=1657.10381727813
  Constant_376.991118430775_bedcf : Constant  Value=376.991118430775
  Product_57b14 : Product
  Product_a9865 : Product
  Blockout_d_vd_bus_8_aabe1 : Outport
  wires:
  Constant_1657.10381727813_58e15/1 -> Product_a9865/1
  Product_57b14/1 -> Add_698bd/2
  Alge_id_bus_8_8b650/1 -> Product_a9865/2
  Constant_376.991118430775_bedcf/1 -> Product_57b14/1
  Product_a9865/1 -> Add_698bd/1
  State_vq_bus_8_643ce/1 -> Product_57b14/2
  Add_698bd/1 -> Blockout_d_vd_bus_8_aabe1/1

== system case8/AC_1/d_vd_bus_9_block ==
  note: d_vd_bus_9 in case8
      | $1564.27849971276\,\mathrm{id}_{\mathrm{bus},9}+376.991118430775\,\mathrm{vq}_{\mathrm{bus},9}$
      | Automatically generated on 2025-10-31 19:30:29 .
  Alge_id_bus_9_9c9c2 : Inport
  State_vq_bus_9_31533 : Inport  Port=2
  Add_d9221 : Sum
  Constant_1564.27849971276_456a9 : Constant  Value=1564.27849971276
  Constant_376.991118430775_8e07e : Constant  Value=376.991118430775
  Product_0f329 : Product
  Product_2ea90 : Product
  Blockout_d_vd_bus_9_f71f4 : Outport
  wires:
  Constant_1564.27849971276_456a9/1 -> Product_0f329/1
  Product_2ea90/1 -> Add_d9221/2
  Alge_id_bus_9_9c9c2/1 -> Product_0f329/2
  Constant_376.991118430775_8e07e/1 -> Product_2ea90/1
  Product_0f329/1 -> Add_d9221/1
  State_vq_bus_9_31533/1 -> Product_2ea90/2
  Add_d9221/1 -> Blockout_d_vd_bus_9_f71f4/1

== system case8/AC_1/d_vq_bus_1_block ==
  note: d_vq_bus_1 in case8
      | $37699111.8430775\,\mathrm{iq}_{\mathrm{bus},1}-376.991118430775\,\mathrm{vd}_{\mathrm{bus},1}$
      | Automatically generated on 2025-10-31 19:30:25 .
  Alge_iq_bus_1_a4066 : Inport
  State_vd_bus_1_06716 : Inport  Port=2
  Constant_376.991118430775_4819b : Constant  Value=376.991118430775
  Constant_37699111.8430775_7e264 : Constant  Value=37699111.8430775
  Product_720f3 : Product
  Product_bca92 : Product
  Subtract_18e60 : Sum  Inputs=+-
  Blockout_d_vq_bus_1_0fecb : Outport
  wires:
  Constant_37699111.8430775_7e264/1 -> Product_720f3/1
  Constant_376.991118430775_4819b/1 -> Product_bca92/1
  Alge_iq_bus_1_a4066/1 -> Product_720f3/2
  State_vd_bus_1_06716/1 -> Product_bca92/2
  Product_720f3/1 -> Subtract_18e60/1
  Product_bca92/1 -> Subtract_18e60/2
  Subtract_18e60/1 -> Blockout_d_vq_bus_1_0fecb/1

== system case8/AC_1/d_vq_bus_2_block ==
  note: d_vq_bus_2 in case8
      | $37699111.8430775\,\mathrm{iq}_{\mathrm{bus},2}-376.991118430775\,\mathrm{vd}_{\mathrm{bus},2}$
      | Automatically generated on 2025-10-31 19:30:25 .
  Alge_iq_bus_2_dfc07 : Inport
  State_vd_bus_2_19465 : Inport  Port=2
  Constant_376.991118430775_56394 : Constant  Value=376.991118430775
  Constant_37699111.8430775_cfeda : Constant  Value=37699111.8430775
  Product_71d40 : Product
  Product_c31e8 : Product
  Subtract_bc64f : Sum  Inputs=+-
  Blockout_d_vq_bus_2_b2178 : Outport
  wires:
  Constant_37699111.8430775_cfeda/1 -> Product_71d40/1
  Constant_376.991118430775_56394/1 -> Product_c31e8/1
  Alge_iq_bus_2_dfc07/1 -> Product_71d40/2
  State_vd_bus_2_19465/1 -> Product_c31e8/2
  Product_71d40/1 -> Subtract_bc64f/1
  Product_c31e8/1 -> Subtract_bc64f/2
  Subtract_bc64f/1 -> Blockout_d_vq_bus_2_b2178/1

== system case8/AC_1/d_vq_bus_3_block ==
  note: d_vq_bus_3 in case8
      | $37699111.8430775\,\mathrm{iq}_{\mathrm{bus},3}-376.991118430775\,\mathrm{vd}_{\mathrm{bus},3}$
      | Automatically generated on 2025-10-31 19:30:26 .
  Alge_iq_bus_3_80dcf : Inport
  State_vd_bus_3_0b9c7 : Inport  Port=2
  Constant_376.991118430775_f38da : Constant  Value=376.991118430775
  Constant_37699111.8430775_63fbd : Constant  Value=37699111.8430775
  Product_26156 : Product
  Product_f1400 : Product
  Subtract_db1e1 : Sum  Inputs=+-
  Blockout_d_vq_bus_3_9ea56 : Outport
  wires:
  Constant_37699111.8430775_63fbd/1 -> Product_f1400/1
  Constant_376.991118430775_f38da/1 -> Product_26156/1
  Alge_iq_bus_3_80dcf/1 -> Product_f1400/2
  State_vd_bus_3_0b9c7/1 -> Product_26156/2
  Product_f1400/1 -> Subtract_db1e1/1
  Product_26156/1 -> Subtract_db1e1/2
  Subtract_db1e1/1 -> Blockout_d_vq_bus_3_9ea56/1

== system case8/AC_1/d_vq_bus_4_block ==
  note: d_vq_bus_4 in case8
      | $2257.43184689087\,\mathrm{iq}_{\mathrm{bus},4}-376.991118430775\,\mathrm{vd}_{\mathrm{bus},4}$
      | Automatically generated on 2025-10-31 19:30:26 .
  Alge_iq_bus_4_a79c6 : Inport
  State_vd_bus_4_25e83 : Inport  Port=2
  Constant_2257.43184689087_ce0e6 : Constant  Value=2257.43184689087
  Constant_376.991118430775_5bf17 : Constant  Value=376.991118430775
  Product_8b440 : Product
  Product_acd74 : Product
  Subtract_13f53 : Sum  Inputs=+-
  Blockout_d_vq_bus_4_4e85a : Outport
  wires:
  Constant_2257.43184689087_ce0e6/1 -> Product_acd74/1
  Constant_376.991118430775_5bf17/1 -> Product_8b440/1
  Alge_iq_bus_4_a79c6/1 -> Product_acd74/2
  State_vd_bus_4_25e83/1 -> Product_8b440/2
  Product_acd74/1 -> Subtract_13f53/1
  Product_8b440/1 -> Subtract_13f53/2
  Subtract_13f53/1 -> Blockout_d_vq_bus_4_4e85a/1

== system case8/AC_1/d_vq_bus_5_block ==
  note: d_vq_bus_5 in case8
      | $1461.2058853906\,\mathrm{iq}_{\mathrm{bus},5}-376.991118430775\,\mathrm{vd}_{\mathrm{bus},5}$
      | Automatically generated on 2025-10-31 19:30:27 .
  Alge_iq_bus_5_593e2 : Inport
  State_vd_bus_5_59ab6 : Inport  Port=2
  Constant_1461.2058853906_0cf44 : Constant  Value=1461.2058853906
  Constant_376.991118430775_836b2 : Constant  Value=376.991118430775
  Product_0c28f : Product
  Product_41487 : Product
  Subtract_cf3b1 : Sum  Inputs=+-
  Blockout_d_vq_bus_5_d199f : Outport
  wires:
  Constant_1461.2058853906_0cf44/1 -> Product_0c28f/1
  Constant_376.991118430775_836b2/1 -> Product_41487/1
  Alge_iq_bus_5_593e2/1 -> Product_0c28f/2
  State_vd_bus_5_59ab6/1 -> Product_41487/2
  Product_0c28f/1 -> Subtract_cf3b1/1
  Product_41487/1 -> Subtract_cf3b1/2
  Subtract_cf3b1/1 -> Blockout_d_vq_bus_5_d199f/1

== system case8/AC_1/d_vq_bus_6_block ==
  note: d_vq_bus_6 in case8
      | $1329.77466818616\,\mathrm{iq}_{\mathrm{bus},6}-376.991118430775\,\mathrm{vd}_{\mathrm{bus},6}$
      | Automatically generated on 2025-10-31 19:30:27 .
  Alge_iq_bus_6_3ba16 : Inport
  State_vd_bus_6_0c589 : Inport  Port=2
  Constant_1329.77466818616_89fd4 : Constant  Value=1329.77466818616
  Constant_376.991118430775_53f35 : Constant  Value=376.991118430775
  Product_22dd7 : Product
  Product_69b74 : Product
  Subtract_8b7e9 : Sum  Inputs=+-
  Blockout_d_vq_bus_6_d63f6 : Outport
  wires:
  Constant_1329.77466818616_89fd4/1 -> Product_69b74/1
  Constant_376.991118430775_53f35/1 -> Product_22dd7/1
  Alge_iq_bus_6_3ba16/1 -> Product_69b74/2
  State_vd_bus_6_0c589/1 -> Product_22dd7/2
  Product_69b74/1 -> Subtract_8b7e9/1
  Product_22dd7/1 -> Subtract_8b7e9/2
  Subtract_8b7e9/1 -> Blockout_d_vq_bus_6_d63f6/1
